simulink model "AUVsim"  (R2018a)
settings: Solver=ode23  StartTime=0.0  StopTime=50  MaxStep=0.1  RelTol=1e-4  EnableMultiTasking=on
undefined symbols (not defined in the file or in its folder): disturbances, disturbonoff, param
settings Model: Creator=tristan  LastModifiedBy=masom
settings DataIOCC: LimitDataPoints=on  SaveFormat=Array  SignalLoggingSaveFormat=ModelDataLogs
settings OptimizationCC: ExpressionDepthLimit=2147483647  LifeSpan=inf
settings DebuggingCC: UnderspecifiedInitializationDetection=Classic  MergeDetectMultiDrivingBlocksExec=none  SolverPrmCheckMsg=warning  StateNameClashWarn=warning  SFUnexpectedBacktrackingDiag=warning  SFNoUnconditionalDefaultTransitionDiag=warning  SFExecutionAtInitializationDiag=none
settings HardwareCC: ProdBitPerPointer=32  ProdBitPerSizeT=32  ProdBitPerPtrDiffT=32  ProdLargestAtomicFloat=None  ProdIntDivRoundTo=Undefined  ProdEndianess=Unspecified  ProdWordSize=32  ProdHWDeviceType=32-bit Generic
settings ModelReferenceCC: PropagateSignalLabelsOutOfModel=off
settings CodeAppCC: StateflowObjectComments=on
settings GRTTargetCC: TargetLangStandard=C89/C90 (ANSI)  GeneratePreprocessorConditionals=Disable all  CombineOutputUpdateFcns=off  GRTInterface=on
settings ConfigComp: CovMetricSettings=dw  CovHtmlReporting=on  CovSaveCumulativeToWorkspaceVar=on  CovSaveSingleToWorkspaceVar=on  CovExternalEMLEnable=off
settings SimscapeCC: SimscapeNormalizeSystem=off
settings ConfigurationSet: Description=SimMechanics 2G

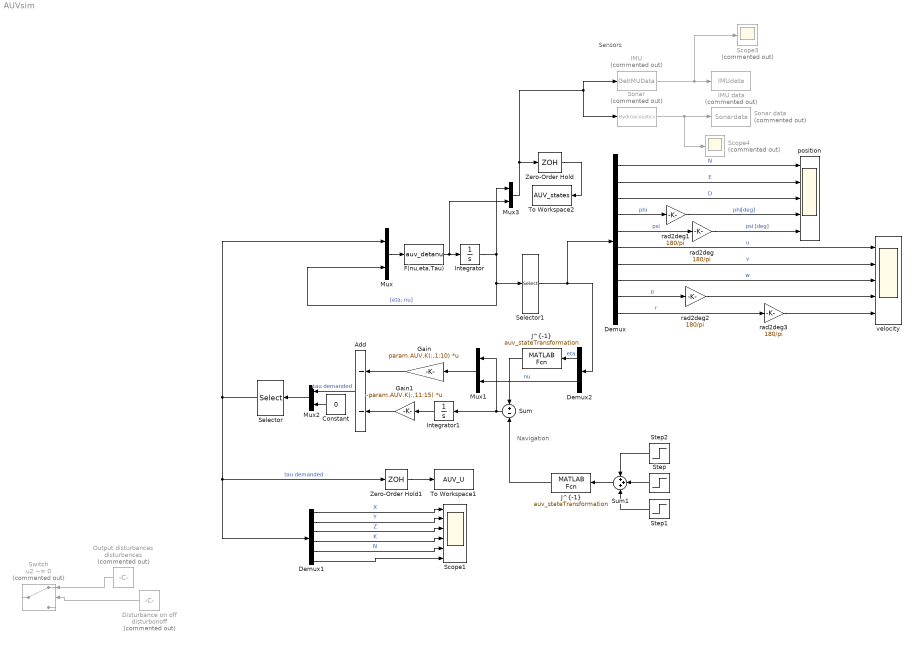
== system AUVsim ==
  note: Sensors
  note: Navigation
  Add : Sum  Inputs=--
  Constant : Constant  Value=0
  Demux : Demux  Outputs=10
  Demux1 : Demux  Outputs=6
  Demux2 : Demux  Outputs=[5,5]
  Disturbance on off : Constant  Commented=on  Value=disturbonoff
  F(nu,eta,Tau) : MATLABFcn  MATLABFcn=auv_detanu  OutputDimensions=12
  Gain : Gain  Gain=param.AUV.K(:,1:10)  Multiplication=Matrix(K*u) (u vector)
  Gain1 : Gain  Gain=-param.AUV.K(:,11:15)  Multiplication=Matrix(K*u) (u vector)
  IMU : MATLABFcn  Commented=on  MATLABFcn=GetIMUData  OutputDimensions=9
  IMU data : ToWorkspace  Commented=on  VariableName=IMUdata  SampleTime=-1
  Integrator : Integrator
  Integrator1 : Integrator
  "J^{-1}" : MATLABFcn  MATLABFcn=auv_stateTransformation  OutputDimensions=5
  "J^{-1} " : MATLABFcn  MATLABFcn=auv_stateTransformation  OutputDimensions=5
  Mux{,1..3} (4 alike) : Mux  Inputs=2
  Output disturbances : Constant  Commented=on  Value=disturbances
  Scope1 : Scope  NumInputPorts=6
  Scope3 : Scope  Commented=on
  Scope4 : Scope  Commented=on
  Selector : Selector  InputPortWidth=6  IndexOptions=Index vector (dialog)  Indices=[1:4,6,5]  OutputSizes=1
  Selector1 : Selector  InputPortWidth=12  IndexOptions=Index vector (dialog)  Indices=[1:4,6:10,12]  OutputSizes=1
  Sonar : MATLABFcn  Commented=on  MATLABFcn=Hydroacoustics  OutputDimensions=8
  Sonar data : ToWorkspace  Commented=on  VariableName=Sonardata  SampleTime=-1
  Step : Step  Time=5  Before=[0, 0, 0, 0, 0]  After=[-30, 0, 0, 0, 0]  SampleTime=0
  Step1 : Step  Time=20  Before=[0, 0, 0, 0, 0]  After=[-15, 0, 0, 0, 0]  SampleTime=0
  Step2 : Step  Time=30  Before=[0, 0, 0, 0, 0]  After=[20, 0, 0, 0, 0]  SampleTime=0
  Sum : Sum  Inputs=+-
  Sum1 : Sum  Inputs=+++
  Switch : Switch  Commented=on  Criteria=u2 ~= 0
  To Workspace1 : ToWorkspace  VariableName=AUV_U  SaveFormat=Timeseries  SampleTime=-1
  To Workspace2 : ToWorkspace  VariableName=AUV_states  SaveFormat=Timeseries  SampleTime=-1
  Zero-Order Hold : ZeroOrderHold  SampleTime=1/param.sensor_sample_rate
  Zero-Order Hold1 : ZeroOrderHold  SampleTime=1/param.sensor_sample_rate
  position : Scope  NumInputPorts=5
  rad2deg{,1..3} (4 alike) : Gain  Gain=180/pi
  velocity : Scope  NumInputPorts=5
  wires:
  Demux1/1 -> Scope1/1  "X"
  Demux1/2 -> Scope1/2  "Y"
  Mux/1 -> F(nu,eta,Tau)/1
  F(nu,eta,Tau)/1 -> Mux3/2, Integrator/1
  Integrator/1 -> Mux3/1, Mux/2, Selector1/1  "[eta; nu]"
  Demux2/2 -> Mux1/2  "nu"
  Sum1/1 -> "J^{-1} "/1
  Demux2/1 -> "J^{-1}"/1  "eta"
  Demux1/4 -> Scope1/4  "K"
  Demux1/3 -> Scope1/3  "Z"
  Demux/5 -> rad2deg/1  "psi"
  Output disturbances/1 -> Switch/1
  Mux1/1 -> Gain/1
  Integrator1/1 -> Gain1/1
  Gain1/1 -> Add/2
  Gain/1 -> Add/1
  Disturbance on off/1 -> Switch/2
  "J^{-1} "/1 -> Sum/2
  "J^{-1}"/1 -> Sum/1
  Selector/1 -> Mux/1, Zero-Order Hold1/1, Demux1/1  "tau demanded"
  Sum/1 -> Integrator1/1, Mux1/1
  Demux/1 -> position/1  "N"
  Demux/2 -> position/2  "E"
  Demux/3 -> position/3  "D"
  rad2deg/1 -> position/5  "psi [deg]"
  rad2deg1/1 -> position/4  "phi[deg]"
  Demux/4 -> rad2deg1/1  "phi"
  Demux/6 -> velocity/1  "u"
  Demux/7 -> velocity/2  "v"
  Demux/8 -> velocity/3  "w"
  Demux/9 -> rad2deg2/1  "p"
  rad2deg2/1 -> velocity/4
  rad2deg3/1 -> velocity/5
  Demux/10 -> rad2deg3/1  "r"
  Demux1/5 -> Scope1/5  "N"
  IMU/1 -> Scope3/1, IMU data/1
  Mux3/1 -> IMU/1, Sonar/1, Zero-Order Hold/1
  Step2/1 -> Sum1/1
  Step/1 -> Sum1/2
  Step1/1 -> Sum1/3
  Sonar/1 -> Scope4/1, Sonar data/1
  Zero-Order Hold/1 -> To Workspace2/1
  Zero-Order Hold1/1 -> To Workspace1/1
  Add/1 -> Mux2/1  "tau demanded"
  Mux2/1 -> Selector/1
  Constant/1 -> Mux2/2
  Selector1/1 -> Demux2/1, Demux/1
  Demux1/6 -> Scope1/6
